simulink model "simhopefeedback"  (R2015b)
settings: Solver=VariableStepAuto  StartTime=0.0  StopTime=10.0  RelTol=1e-3
settings Model: Creator=29118  LastModifiedBy=朱明菲

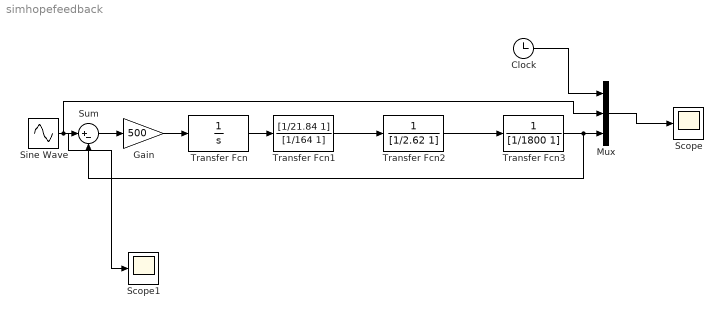
== system simhopefeedback ==
  Clock : Clock
  Gain : Gain  Gain=500
  Mux : Mux  Inputs=3
  Scope : Scope
  Scope1 : Scope
  Sine Wave : Sin  SampleTime=0
  Sum : Sum  Inputs=|+-
  Transfer Fcn : TransferFcn  Denominator=[1 0]
  Transfer Fcn1 : TransferFcn  Numerator=[1/21.84 1]  Denominator=[1/164 1]
  Transfer Fcn2 : TransferFcn  Denominator=[1/2.62 1]
  Transfer Fcn3 : TransferFcn  Denominator=[1/1800 1]
  wires:
  Transfer Fcn/1 -> Transfer Fcn1/1
  Transfer Fcn1/1 -> Transfer Fcn2/1
  Transfer Fcn2/1 -> Transfer Fcn3/1
  Gain/1 -> Transfer Fcn/1
  Sine Wave/1 -> Mux/2, Scope1/1, Sum/1
  Sum/1 -> Gain/1
  Mux/1 -> Scope/1
  Transfer Fcn3/1 -> Mux/3, Sum/2
  Clock/1 -> Mux/1
